simulink model "PrimeiraOrdemQuadrado"  (R2015a)
settings: Solver=ode45  StartTime=0.0  StopTime=10  FixedStep=0.00001  RelTol=1e-5
settings Model: Creator=user  LastModifiedBy=user
settings SolverCC: ZeroCrossAlgorithm=Adaptive
settings DebuggingCC: UnderspecifiedInitializationDetection=Classic

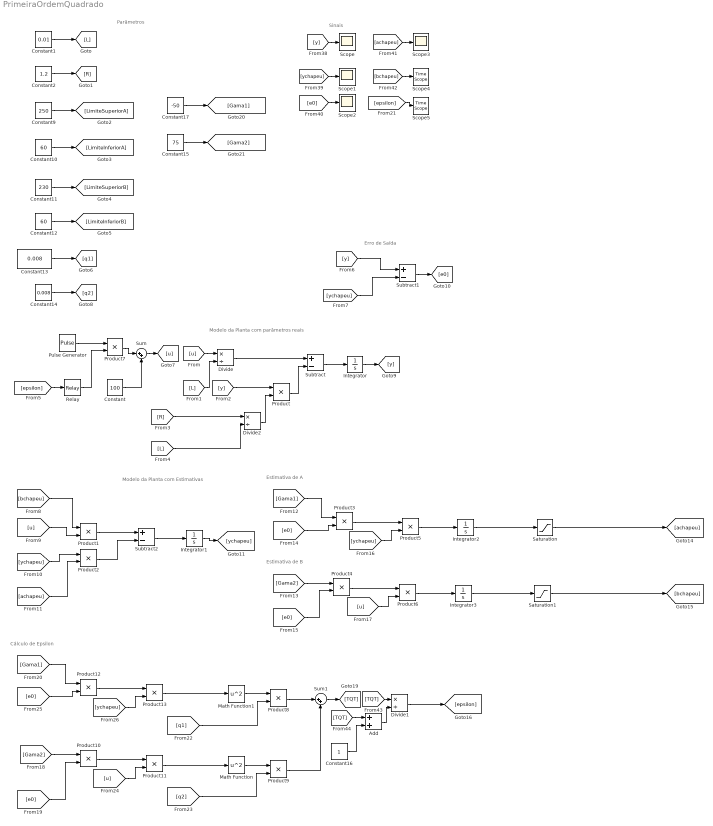
== system PrimeiraOrdemQuadrado ==
  note: Cálculo de Epsilon
  note: Estimativa de B
  note: Estimativa de A
  note: Modelo da Planta com Estimativas
  note: Modelo da Planta com parâmetros reais
  note: Erro de Saída
  note: Parâmetros
  note: Sinais
  Add : Sum  AccumDataTypeStr=double
  Constant : Constant  Value=100
  Constant1 : Constant  Value=0.01
  Constant10 : Constant  Value=60
  Constant11 : Constant  Value=230
  Constant12 : Constant  Value=60
  Constant13 : Constant  Value=0.008
  Constant14 : Constant  Value=0.008
  Constant15 : Constant  Value=75
  Constant16 : Constant
  Constant17 : Constant  Value=-50
  Constant2 : Constant  Value=1.2
  Constant9 : Constant  Value=250
  Divide : Product  Inputs=*/
  Divide1 : Product  Inputs=*/  OutDataTypeStr=double
  Divide2 : Product  Inputs=*/
  Integrator : Integrator
  Integrator1 : Integrator
  Integrator2 : Integrator  InitialCondition=70
  Integrator3 : Integrator  InitialCondition=80
  Math Function : Math  Operator=square  SaturateOnIntegerOverflow=on
  Math Function1 : Math  Operator=square  SaturateOnIntegerOverflow=on
  Product{,1..13} (14 alike) : Product
  Pulse Generator : DiscretePulseGenerator  PulseType=Time based  Amplitude=100  Period=0.1  PulseWidth=50
  Relay : Relay  OnSwitchValue=0.5  OffSwitchValue=0.5
  Saturation : Saturate  UpperLimit=500  LowerLimit=1
  Saturation1 : Saturate  UpperLimit=300  LowerLimit=1
  Scope{,1..3} (4 alike) : Scope
      Scope settings: YMin=80  YMax=170
      Scope1 settings: YMin=80  YMax=170  SampleInput=on
      Scope2 settings: YMin=-0.35  YMax=0.3  SaveName=ScopeData2  SampleInput=on
      Scope3 settings: YMin=113.818  YMax=113.853  SaveName=ScopeData3  SampleInput=on
  Scope4 : TimeScope
  Scope5 : TimeScope
  Subtract : Sum  Inputs=+-
  Subtract1 : Sum  Inputs=+-
  Subtract2 : Sum  Inputs=+-
  Sum : Sum  Inputs=|++
  Sum1 : Sum  Inputs=|++
  wires:
  Constant/1 -> Sum/2
  [L] -> Divide/2
  Divide2/1 -> Product/2
  [L] -> Divide2/2
  [R] -> Divide2/1
  Product/1 -> Subtract/2
  Divide/1 -> Subtract/1
  Subtract/1 -> Integrator/1
  Integrator/1 -> [y]
  [y] -> Product/1
  Sum/1 -> [u]
  [u] -> Divide/1
  [y] -> Subtract1/1
  [ychapeu] -> Subtract1/2
  Subtract1/1 -> [e0]
  Constant1/1 -> [L]
  Constant2/1 -> [R]
  Product1/1 -> Subtract2/1
  Subtract2/1 -> Integrator1/1
  Product2/1 -> Subtract2/2
  [achapeu] -> Product2/2
  [ychapeu] -> Product2/1
  [u] -> Product1/2
  [bchapeu] -> Product1/1
  Integrator1/1 -> [ychapeu]
  [e0] -> Product3/2
  [Gama1] -> Product3/1
  [Gama2] -> Product4/1
  [e0] -> Product4/2
  Product4/1 -> Product6/1
  Product3/1 -> Product5/1
  [ychapeu] -> Product5/2
  [u] -> Product6/2
  Product5/1 -> Integrator2/1
  Product6/1 -> Integrator3/1
  Integrator3/1 -> Saturation1/1
  Integrator2/1 -> Saturation/1
  Product7/1 -> Sum/1
  Pulse Generator/1 -> Product7/1
  Product11/1 -> Math Function/1
  Product13/1 -> Math Function1/1
  Math Function1/1 -> Product8/1
  Math Function/1 -> Product9/1
  [q1] -> Product8/2
  [q2] -> Product9/2
  Product9/1 -> Sum1/2
  Product8/1 -> Sum1/1
  Constant9/1 -> [LimiteSuperiorA]
  Constant10/1 -> [LimiteInferiorA]
  Constant11/1 -> [LimiteSuperiorB]
  Constant12/1 -> [LimiteInferiorB]
  Constant13/1 -> [q1]
  Constant14/1 -> [q2]
  [y] -> Scope/1
  [ychapeu] -> Scope1/1
  [e0] -> Scope2/1
  [achapeu] -> Scope3/1
  [bchapeu] -> Scope4/1
  Constant17/1 -> [Gama1]
  Constant15/1 -> [Gama2]
  Divide1/1 -> [epsilon]
  Add/1 -> Divide1/2
  Constant16/1 -> Add/2
  Sum1/1 -> [TQT]
  [TQT] -> Divide1/1
  [TQT] -> Add/1
  [epsilon] -> Relay/1
  Saturation/1 -> [achapeu]
  Saturation1/1 -> [bchapeu]
  [Gama2] -> Product10/1
  [e0] -> Product10/2
  Product10/1 -> Product11/1
  [u] -> Product11/2
  [e0] -> Product12/2
  [Gama1] -> Product12/1
  Product12/1 -> Product13/1
  [ychapeu] -> Product13/2
  Relay/1 -> Product7/2
  [epsilon] -> Scope5/1
